simulink model "generating_sine_for_pwmsignal"  (R2013a)
settings: Solver=ode45  StartTime=0.0  StopTime=1  MaxStep=0.00001  RelTol=1e-6  AbsTol=1e-3
libraries: powerlib x8, simulink x4
settings Model: BufferReuse=off  Creator=boby  LastModifiedBy=boby
settings SolverCC: ShapePreserveControl=EnableAll  ZeroCrossControl=DisableAll  ZeroCrossAlgorithm=Adaptive
settings OptimizationCC: BlockReduction=off  InlineParams=on  BufferReuse=off

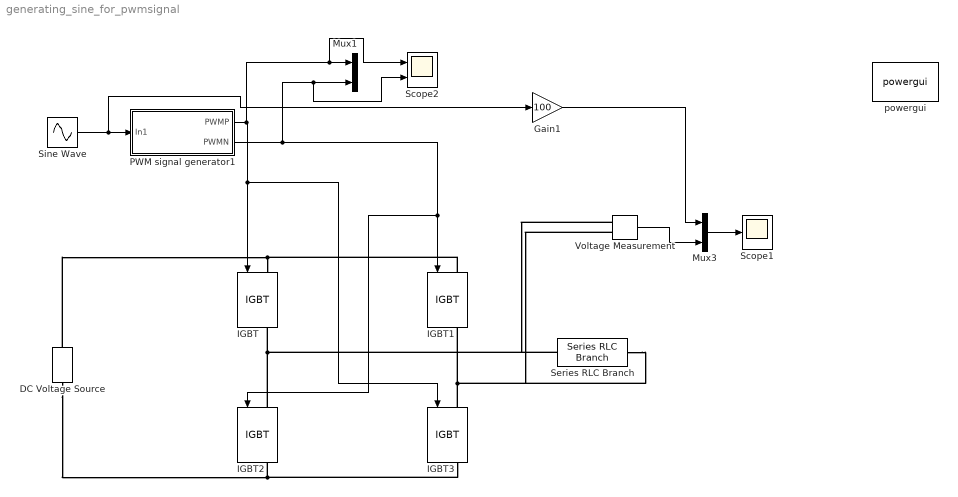
== system generating_sine_for_pwmsignal ==
  DC Voltage Source : powerlib/Electrical Sources/DC Voltage Source  Amplitude=100  Measurements=None
  Gain1 : Gain  Gain=100
  IGBT{,1..3} (4 alike) : powerlib/Power Electronics/IGBT  Ron=0.001  Lon=0  Vf=1  Tf=1e-6  Tt=2e-6  IC=0  Rs=1e5  Cs=inf  Measurements=on
  Mux1 : Mux  Inputs=2
  Mux3 : Mux  Inputs=2
  PWM signal generator1 : Subsystem
  Scope1 : Scope
      settings: SaveName=ScopeData5
  Scope2 : Scope  NumInputPorts=2
      settings: YMin=-5~-5  YMax=5~5  SaveName=ScopeData6
  Series RLC Branch : powerlib/Elements/Series RLC Branch  LConnTagsString=__new0  RConnTagsString=__new0  BranchType=R  Resistance=1  Inductance=1e-3  SetiL0=off  InitialCurrent=0  Capacitance=1e-6  Setx0=off  InitialVoltage=0  Measurements=None
  Sine Wave : Sin  Frequency=2*pi*50  SampleTime=0
  Voltage Measurement : powerlib/Measurements/Voltage Measurement  PhasorSimulation=off  OutputType=Complex  PSBequivalent=0
  powergui : powerlib/powergui  Priority=1  SimulationMode=Continuous  SolverType=Tustin  SampleTime=50e-6  frequency=60  SPID=off  DisableSnubberDevices=off  DisableRonSwitches=off  DisableVfSwitches=off  SwTol=0  Interpol=off  DisplayEquations=off  frequencyindice=0  Pbase=100e6  ErrMax=1e-4  Iterations=50  UnitsV=kV  UnitsW=MW  FunctionMessages=off  echomessages=off  HookPort=off  EnableUseOfTLC=off  x0status=blocks  RestoreLinks=warning  ResistiveCurrentMeasurement=off  Frange=[0:2:500]  Ylog=off  Xlog=on  ShowGrid=off  save=off  variable=ZData  ZoomFFT=off  StartTime=0.0  cycles=1  DisplayStyle=1  fundamental=60  FreqAxis=off  MaxFrequency=1000  frequencyindicesteady=1  RmsSteady=1  display=off  Ts=0  methode=off
  wires:
  Sine Wave/1 -> Gain1/1, PWM signal generator1/1(In1)
  Mux3/1 -> Scope1/1
  Voltage Measurement/1 -> Mux3/2
  PWM signal generator1/1(PWMP) -> Scope2/1, Mux1/1, IGBT3/1, IGBT/1
  PWM signal generator1/2(PWMN) -> Scope2/2, Mux1/2, IGBT2/1, IGBT1/1
  Gain1/1 -> Mux3/1
  connections:
  DC Voltage Source/RConn1 -- IGBT1/LConn1 -- IGBT/LConn1
  DC Voltage Source/LConn1 -- IGBT3/RConn1 -- IGBT2/RConn1
  IGBT2/LConn1 -- Voltage Measurement/LConn1 -- Series RLC Branch/LConn1 -- IGBT/RConn1
  IGBT3/LConn1 -- Voltage Measurement/LConn2 -- Series RLC Branch/RConn1 -- IGBT1/RConn1

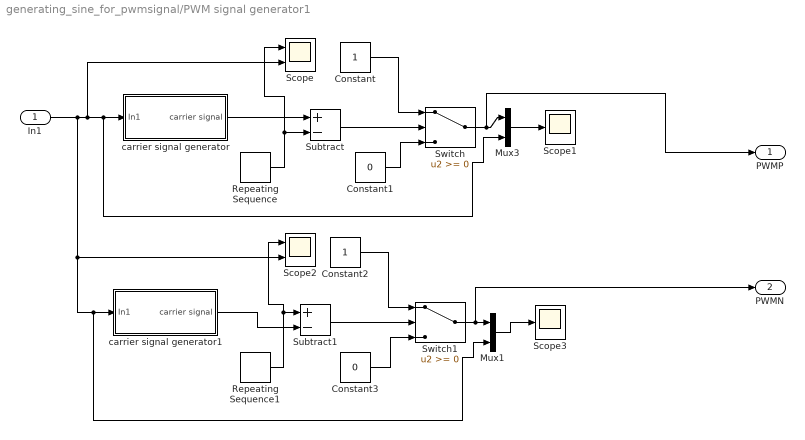
== system generating_sine_for_pwmsignal/PWM signal generator1 ==
  In1 : Inport
  Constant : Constant
  Constant1 : Constant  Value=0
  Constant2 : Constant
  Constant3 : Constant  Value=0
  Mux1 : Mux  Inputs=2
  Mux3 : Mux  Inputs=2
  Repeating Sequence : simulink/Sources/Repeating Sequence  rep_seq_t=[0 0.0001 0.0003 0.0004]  rep_seq_y=[0 0.8 -0.8 0]
  Repeating Sequence1 : simulink/Sources/Repeating Sequence  rep_seq_t=[0 0.0001 0.0003 0.0004]  rep_seq_y=[0 0.8 -0.8 0]
  Scope : Scope  NumInputPorts=2
      settings: YMin=-5~-5  YMax=5~5
  Scope1 : Scope
      settings: SaveName=ScopeData2
  Scope2 : Scope  NumInputPorts=2
      settings: YMin=-5~-5  YMax=5~5  SaveName=ScopeData3
  Scope3 : Scope
      settings: SaveName=ScopeData4
  Subtract : Sum  Inputs=+-
  Subtract1 : Sum  Inputs=+-
  Switch : Switch
  Switch1 : Switch
  carrier signal generator : Subsystem
  carrier signal generator1 : Subsystem
  PWMP : Outport
  PWMN : Outport  Port=2
  wires:
  carrier signal generator/1(carrier signal) -> Subtract/1
  Repeating Sequence/1 -> Scope/1, Subtract/2
  Subtract/1 -> Switch/2
  Constant/1 -> Switch/1
  Constant1/1 -> Switch/3
  Switch/1 -> PWMP/1, Mux3/1
  Mux3/1 -> Scope1/1
  In1/1 -> Mux1/2, carrier signal generator1/1(In1), Scope2/2, Scope/2, Mux3/2, carrier signal generator/1(In1)
  Subtract1/1 -> Switch1/2
  Constant2/1 -> Switch1/1
  Constant3/1 -> Switch1/3
  Switch1/1 -> PWMN/1, Mux1/1
  Mux1/1 -> Scope3/1
  carrier signal generator1/1(carrier signal) -> Subtract1/2
  Repeating Sequence1/1 -> Scope2/1, Subtract1/1

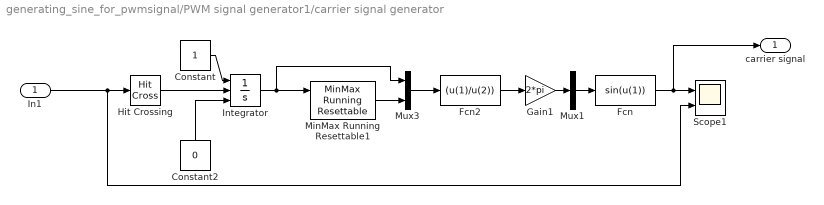
== system generating_sine_for_pwmsignal/PWM signal generator1/carrier signal generator ==
  In1 : Inport
  Constant : Constant
  Constant2 : Constant  Value=0
  Fcn : Fcn  Expr=sin(u(1))
  Fcn2 : Fcn  Expr=(u(1)/u(2))
  Gain1 : Gain  Gain=2*pi
  Hit Crossing : HitCross  HitCrossingDirection=rising
  Integrator : Integrator  ExternalReset=rising  InitialConditionSource=external
  MinMax Running Resettable1 : simulink/Math Operations/MinMax Running Resettable  Function=max  vinit=0.0
  Mux1 : Mux  Inputs=1
  Mux3 : Mux  Inputs=2
  Scope1 : Scope  NumInputPorts=2
      settings: YMin=-5~-5  YMax=5~5
  carrier signal : Outport
  wires:
  Constant/1 -> Integrator/1
  Mux1/1 -> Fcn/1
  Hit Crossing/1 -> Integrator/2
  Constant2/1 -> Integrator/3
  Integrator/1 -> Mux3/1, MinMax Running Resettable1/1
  MinMax Running Resettable1/1 -> Mux3/2
  Fcn2/1 -> Gain1/1
  Gain1/1 -> Mux1/1
  Fcn/1 -> carrier signal/1, Scope1/1
  In1/1 -> Scope1/2, Hit Crossing/1
  Mux3/1 -> Fcn2/1

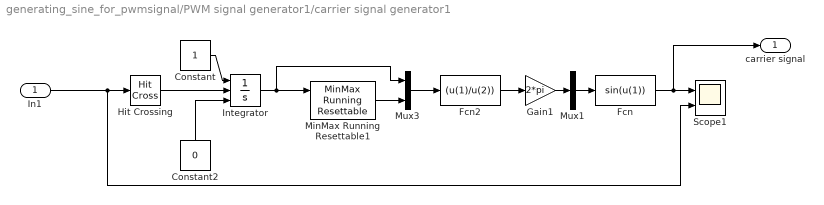
== system generating_sine_for_pwmsignal/PWM signal generator1/carrier signal generator1 ==
  In1 : Inport
  Constant : Constant
  Constant2 : Constant  Value=0
  Fcn : Fcn  Expr=sin(u(1))
  Fcn2 : Fcn  Expr=(u(1)/u(2))
  Gain1 : Gain  Gain=2*pi
  Hit Crossing : HitCross  HitCrossingDirection=rising
  Integrator : Integrator  ExternalReset=rising  InitialConditionSource=external
  MinMax Running Resettable1 : simulink/Math Operations/MinMax Running Resettable  Function=max  vinit=0.0
  Mux1 : Mux  Inputs=1
  Mux3 : Mux  Inputs=2
  Scope1 : Scope  NumInputPorts=2
      settings: YMin=-5~-5  YMax=5~5
  carrier signal : Outport
  wires:
  Constant/1 -> Integrator/1
  Mux1/1 -> Fcn/1
  Hit Crossing/1 -> Integrator/2
  Constant2/1 -> Integrator/3
  Integrator/1 -> Mux3/1, MinMax Running Resettable1/1
  MinMax Running Resettable1/1 -> Mux3/2
  Fcn2/1 -> Gain1/1
  Gain1/1 -> Mux1/1
  Fcn/1 -> carrier signal/1, Scope1/1
  In1/1 -> Scope1/2, Hit Crossing/1
  Mux3/1 -> Fcn2/1
